simulink model "Double_mass_spring_model"  (R2018b)
settings: Solver=ode4  StartTime=0.0  StopTime=100  FixedStep=0.005  RelTol=1e-3
undefined symbols (not defined in the file or in its folder): c1_main, c1_nose, c2_main, c2_nose, k1_main, k1_nose, k2_main, k2_nose, m1, m2, m3
settings Model: Creator=e805358  LastModifiedBy=e805358
settings DataIOCC: ExternalInput=[t]  SaveState=on  SignalLogging=off  DSMLogging=off

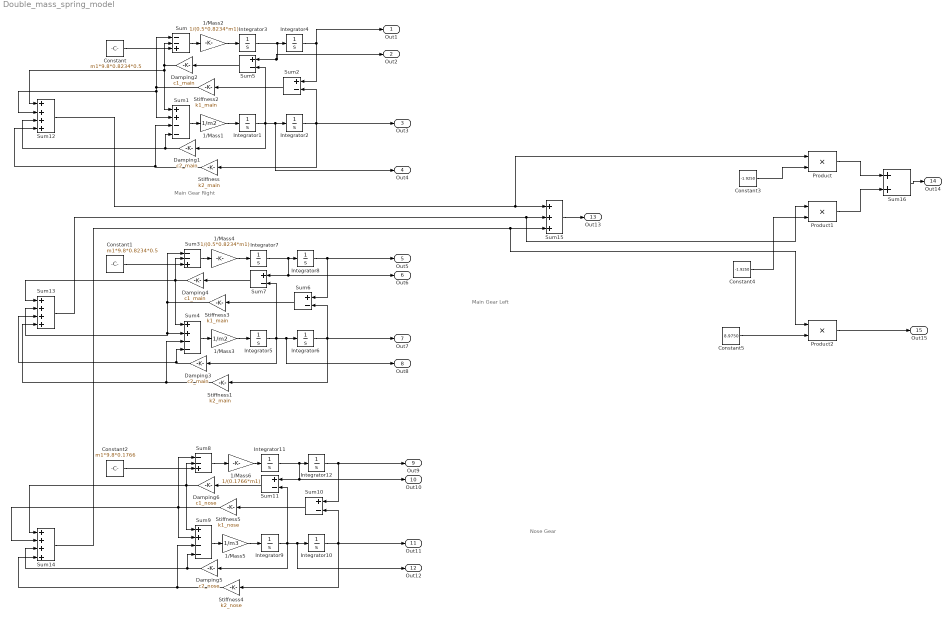
== system Double_mass_spring_model ==
  note: Main Gear Right
  note: Main Gear Left
  note: Nose Gear
  1/Mass1 : Gain  Gain=1/m2  SaturateOnIntegerOverflow=on  OutDataTypeStr=Inherit: Same as input  ParamDataTypeStr=Inherit: Same as input
  1/Mass2 : Gain  Gain=1/(0.5*0.8234*m1)  SaturateOnIntegerOverflow=on  OutDataTypeStr=Inherit: Same as input  ParamDataTypeStr=Inherit: Same as input
  1/Mass3 : Gain  Gain=1/m2  SaturateOnIntegerOverflow=on  OutDataTypeStr=Inherit: Same as input  ParamDataTypeStr=Inherit: Same as input
  1/Mass4 : Gain  Gain=1/(0.5*0.8234*m1)  SaturateOnIntegerOverflow=on  OutDataTypeStr=Inherit: Same as input  ParamDataTypeStr=Inherit: Same as input
  1/Mass5 : Gain  Gain=1/m3  SaturateOnIntegerOverflow=on  OutDataTypeStr=Inherit: Same as input  ParamDataTypeStr=Inherit: Same as input
  1/Mass6 : Gain  Gain=1/(0.1766*m1)  SaturateOnIntegerOverflow=on  OutDataTypeStr=Inherit: Same as input  ParamDataTypeStr=Inherit: Same as input
  Constant : Constant  Value=m1*9.8*0.8234*0.5
  Constant1 : Constant  Value=m1*9.8*0.8234*0.5
  Constant2 : Constant  Value=m1*9.8*0.1766
  Constant3 : Constant  Value=-1.9250
  Constant4 : Constant  Value=-1.9250
  Constant5 : Constant  Value=8.9750
  Damping1 : Gain  Gain=c2_main  SaturateOnIntegerOverflow=on  OutDataTypeStr=Inherit: Same as input  ParamDataTypeStr=Inherit: Same as input
  Damping2 : Gain  Gain=c1_main  SaturateOnIntegerOverflow=on  OutDataTypeStr=Inherit: Same as input  ParamDataTypeStr=Inherit: Same as input
  Damping3 : Gain  Gain=c2_main  SaturateOnIntegerOverflow=on  OutDataTypeStr=Inherit: Same as input  ParamDataTypeStr=Inherit: Same as input
  Damping4 : Gain  Gain=c1_main  SaturateOnIntegerOverflow=on  OutDataTypeStr=Inherit: Same as input  ParamDataTypeStr=Inherit: Same as input
  Damping5 : Gain  Gain=c2_nose  SaturateOnIntegerOverflow=on  OutDataTypeStr=Inherit: Same as input  ParamDataTypeStr=Inherit: Same as input
  Damping6 : Gain  Gain=c1_nose  SaturateOnIntegerOverflow=on  OutDataTypeStr=Inherit: Same as input  ParamDataTypeStr=Inherit: Same as input
  Integrator1 : Integrator  ContinuousStateAttributes='MGR3'
  Integrator10 : Integrator  ContinuousStateAttributes='NG4'
      settings: AttributesFormatString=x0 = %<InitialCondition> m
  Integrator11 : Integrator  ContinuousStateAttributes='NG1'
  Integrator12 : Integrator  ContinuousStateAttributes='NG2'
      settings: AttributesFormatString=x0 = %<InitialCondition> m
  Integrator2 : Integrator  ContinuousStateAttributes='MGR4'
      settings: AttributesFormatString=x0 = %<InitialCondition> m
  Integrator3 : Integrator  ContinuousStateAttributes='MGR1'
  Integrator4 : Integrator  ContinuousStateAttributes='MGR2'
      settings: AttributesFormatString=x0 = %<InitialCondition> m
  Integrator5 : Integrator  ContinuousStateAttributes='MGL3'
  Integrator6 : Integrator  ContinuousStateAttributes='MGL4'
      settings: AttributesFormatString=x0 = %<InitialCondition> m
  Integrator7 : Integrator  ContinuousStateAttributes='MGL1'
  Integrator8 : Integrator  ContinuousStateAttributes='MGL2'
      settings: AttributesFormatString=x0 = %<InitialCondition> m
  Integrator9 : Integrator  ContinuousStateAttributes='NG3'
  Product : Product
  Product1 : Product
  Product2 : Product
  Stiffness : Gain  Gain=k2_main  SaturateOnIntegerOverflow=on  OutDataTypeStr=Inherit: Same as input  ParamDataTypeStr=Inherit: Same as input
  Stiffness1 : Gain  Gain=k2_main  SaturateOnIntegerOverflow=on  OutDataTypeStr=Inherit: Same as input  ParamDataTypeStr=Inherit: Same as input
  Stiffness2 : Gain  Gain=k1_main  SaturateOnIntegerOverflow=on  OutDataTypeStr=Inherit: Same as input  ParamDataTypeStr=Inherit: Same as input
  Stiffness3 : Gain  Gain=k1_main  SaturateOnIntegerOverflow=on  OutDataTypeStr=Inherit: Same as input  ParamDataTypeStr=Inherit: Same as input
  Stiffness4 : Gain  Gain=k2_nose  SaturateOnIntegerOverflow=on  OutDataTypeStr=Inherit: Same as input  ParamDataTypeStr=Inherit: Same as input
  Stiffness5 : Gain  Gain=k1_nose  SaturateOnIntegerOverflow=on  OutDataTypeStr=Inherit: Same as input  ParamDataTypeStr=Inherit: Same as input
  Sum : Sum  Inputs=--+  SaturateOnIntegerOverflow=on  InputSameDT=on  OutDataTypeStr=Inherit: Same as first input
  Sum1 : Sum  Inputs=++--  SaturateOnIntegerOverflow=on  InputSameDT=on  OutDataTypeStr=Inherit: Same as first input
  Sum{2,5..7,10..11} (6 alike) : Sum  Inputs=+-  SaturateOnIntegerOverflow=on  InputSameDT=on  OutDataTypeStr=Inherit: Same as first input
  Sum12 : Sum  Inputs=++++  SaturateOnIntegerOverflow=on  InputSameDT=on  OutDataTypeStr=Inherit: Same as first input
  Sum13 : Sum  Inputs=++++  SaturateOnIntegerOverflow=on  InputSameDT=on  OutDataTypeStr=Inherit: Same as first input
  Sum14 : Sum  Inputs=++++  SaturateOnIntegerOverflow=on  InputSameDT=on  OutDataTypeStr=Inherit: Same as first input
  Sum15 : Sum  Inputs=+++  SaturateOnIntegerOverflow=on  InputSameDT=on  OutDataTypeStr=Inherit: Same as first input
  Sum16 : Sum  SaturateOnIntegerOverflow=on  InputSameDT=on  OutDataTypeStr=Inherit: Same as first input
  Sum3 : Sum  Inputs=--+  SaturateOnIntegerOverflow=on  InputSameDT=on  OutDataTypeStr=Inherit: Same as first input
  Sum4 : Sum  Inputs=++--  SaturateOnIntegerOverflow=on  InputSameDT=on  OutDataTypeStr=Inherit: Same as first input
  Sum8 : Sum  Inputs=--+  SaturateOnIntegerOverflow=on  InputSameDT=on  OutDataTypeStr=Inherit: Same as first input
  Sum9 : Sum  Inputs=++--  SaturateOnIntegerOverflow=on  InputSameDT=on  OutDataTypeStr=Inherit: Same as first input
  Out1 : Outport
  Out2 : Outport  Port=2
  Out3 : Outport  Port=3
  Out4 : Outport  Port=4
  Out5 : Outport  Port=5
  Out6 : Outport  Port=6
  Out7 : Outport  Port=7
  Out8 : Outport  Port=8
  Out9 : Outport  Port=9
  Out10 : Outport  Port=10
  Out11 : Outport  Port=11
  Out12 : Outport  Port=12
  Out13 : Outport  Port=13
  Out14 : Outport  Port=14
  Out15 : Outport  Port=15
  wires:
  Sum/1 -> 1/Mass2/1
  Integrator1/1 -> Sum5/2, Out4/1, Integrator2/1, Damping1/1
  Damping1/1 -> Sum12/3, Sum1/4
  Stiffness/1 -> Sum12/4, Sum1/3
  Stiffness2/1 -> Sum12/2, Sum1/2, Sum/1
  Integrator2/1 -> Out3/1, Sum2/2, Stiffness/1
  Sum1/1 -> 1/Mass1/1
  Damping2/1 -> Sum/2, Sum12/1, Sum1/1
  Integrator4/1 -> Out1/1, Sum2/1
  1/Mass1/1 -> Integrator1/1
  Sum2/1 -> Stiffness2/1
  1/Mass2/1 -> Integrator3/1
  Sum5/1 -> Damping2/1
  Integrator3/1 -> Out2/1, Sum5/1, Integrator4/1
  Stiffness3/1 -> Sum13/2, Sum4/2, Sum3/1
  Stiffness1/1 -> Sum13/4, Sum4/3
  Damping3/1 -> Sum13/3, Sum4/4
  Sum3/1 -> 1/Mass4/1
  Sum7/1 -> Damping4/1
  Integrator7/1 -> Sum7/1, Out6/1, Integrator8/1
  1/Mass4/1 -> Integrator7/1
  Sum6/1 -> Stiffness3/1
  1/Mass3/1 -> Integrator5/1
  Integrator8/1 -> Out5/1, Sum6/1
  Damping4/1 -> Sum4/1, Sum13/1, Sum3/2
  Integrator6/1 -> Out7/1, Sum6/2, Stiffness1/1
  Sum4/1 -> 1/Mass3/1
  Integrator5/1 -> Sum7/2, Out8/1, Integrator6/1, Damping3/1
  1/Mass5/1 -> Integrator9/1
  Sum10/1 -> Stiffness5/1
  1/Mass6/1 -> Integrator11/1
  Integrator11/1 -> Sum11/1, Out10/1, Integrator12/1
  Sum8/1 -> 1/Mass6/1
  Stiffness4/1 -> Sum14/4, Sum9/3
  Stiffness5/1 -> Sum9/2, Sum14/2, Sum8/1
  Sum11/1 -> Damping6/1
  Sum9/1 -> 1/Mass5/1
  Damping6/1 -> Sum14/1, Sum8/2, Sum9/1
  Integrator10/1 -> Out11/1, Sum10/2, Stiffness4/1
  Integrator9/1 -> Sum11/2, Out12/1, Integrator10/1, Damping5/1
  Damping5/1 -> Sum14/3, Sum9/4
  Integrator12/1 -> Out9/1, Sum10/1
  Sum12/1 -> Product/1, Sum15/1
  Sum13/1 -> Product1/1, Sum15/2
  Sum14/1 -> Product2/1, Sum15/3
  Sum15/1 -> Out13/1
  Constant3/1 -> Product/2
  Constant4/1 -> Product1/2
  Product/1 -> Sum16/1
  Product1/1 -> Sum16/2
  Sum16/1 -> Out14/1
  Constant5/1 -> Product2/2
  Product2/1 -> Out15/1
  Constant/1 -> Sum/3
  Constant1/1 -> Sum3/3
  Constant2/1 -> Sum8/3
